simulink model "HW_1_v2_2019a_signal_builder"  (R2019a)
settings: Solver=VariableStepAuto  StartTime=0.0  StopTime=70  RelTol=1e-12
model workspace (MAT data in the model file):
  d_tar = 20
values from neighbouring files (symbols this model uses):
  d_0 = 8    [acc1.m]
  t_H_tar = 1    [acc1.m]
  v_H0 = 28    [acc1.m]
  v_L0 = 36    [acc1.m]
  v_tar = 36    [acc1.m]
  x_H0 = 0    [acc1.m]
  x_L0 = 50    [acc1.m]
undefined symbols (not defined in the file or in its folder): sigbuilder_block
libraries: cstblocks x3, fl_lib x1
settings Model: Creator=jake  LastModifiedBy=jake
settings DebuggingCC: SFMachineParentedDataDiag=error

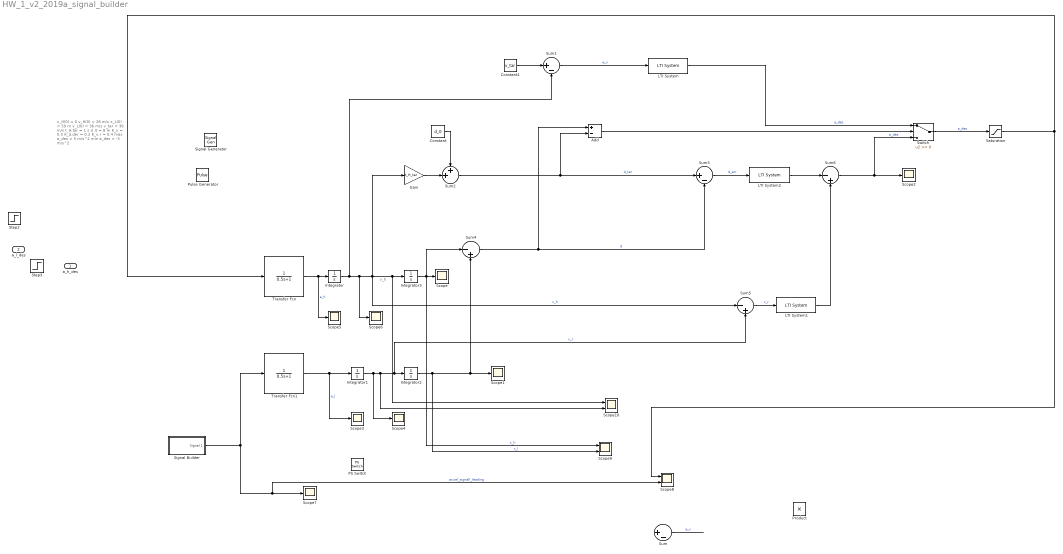
== system HW_1_v2_2019a_signal_builder ==
  note: x_H(0) = 0
      | v_H(0) = 28 m/s
      |
      | x_L(0) = 50 m
      | v_L(0) = 36 m/s
      |
      | v_tar = 36 m/s
      | t_H,tar = 1 s
      | d_0 = 8 m
      |
      | K_v = 0.5
      | K_d,der = 0.2
      | K_v,r = 0.4
      |
      | max a_des = 5 m/s^2
      | min a_des = -3 m/s^2
  note: v_h
  a_h_des : Inport
  a_l_des : Inport  Port=2
  Add : Sum  Inputs=+-
  Constant : Constant  Value=d_0
  Constant1 : Constant  Value=v_tar
  Gain : Gain  Gain=t_H_tar
  Integrator : Integrator  InitialCondition=v_H0
  Integrator1 : Integrator  InitialCondition=v_L0
  Integrator2 : Integrator  InitialCondition=x_L0
  Integrator3 : Integrator  InitialCondition=x_H0
  LTI System : cstblocks/LTI System  sys=K_v  IC=[]
  LTI System1 : cstblocks/LTI System  sys=K_v_r  IC=[]
  LTI System2 : cstblocks/LTI System  sys=K_d_err  IC=[]
  PS Switch : fl_lib/Physical Signals/Nonlinear Operators/PS Switch  Threshold=0.5
      settings: SourceProductBaseCode=SS  InternalSimscapePortConfiguration="{\"Bottom\":[],\"Left\":[{\"id\":\"I1\",\"label\":\"\",\"type\":\"input\"},{\"id\":\"I2\",\"label\":\"\",\"type\":\"input\"},{\"id\":\"I3\",\"label\":\"\",\"type\":\"input\"}],\"Right\":[{\"id\":\"O\",\"label\":\"\",\"type\":\"output\"}],\"Top\":[]}"
  Product : Product
  Pulse Generator : DiscretePulseGenerator  PulseType=Time based  Period=10  PulseWidth=5
  Saturation : Saturate  UpperLimit=5  LowerLimit=-3
  Scope{,1..7} (8 alike) : Scope
  Scope10 : Scope  NumInputPorts=2
  Scope8 : Scope  NumInputPorts=2
  Scope9 : Scope  NumInputPorts=2
  Signal Generator : SignalGenerator  Units=rad/sec
  Signal Builder : Subsystem  Tag=STV Subsys  LoadFcn=sigbuilder_block('load');  StartFcn=sigbuilder_block('start');  StopFcn=sigbuilder_block('stop');  ClipboardFcn=sigbuilder_block('clipboard');  mask(Sigbuilder block){tuvar=[0:10]}
      mask help: Simulink:masks:SigbuilderBlock_MD
      mask init:
      | if ~strcmp(get_param(bdroot(gcbh),'SimulationStatus'),'stopped') tuvar = sigbuilder_block('maskInit'); end
      settings: CopyFcn=sigbuilder_block('copy');  DeleteFcn=sigbuilder_block('delete');  ModelCloseFcn=sigbuilder_block('modelClose');  PreSaveFcn=sigbuilder_block('preSave');  PauseFcn=sigbuilder_block('pause');  ContinueFcn=sigbuilder_block('continue');  NameChangeFcn=sigbuilder_block('namechange');  OpenFcn=sigbuilder_block('open',[553.5 167.25 843.75 498.75 ]);  CloseFcn=sigbuilder_block('close');
      mask Display: plot(0, 0, 100, 100,[2, 2, 32, 32, 2], [68, 8, 8, 68, 68],[32, 2], [38, 38], [32, 19, 2],[53, 60, 44], [32, 17, 17, 2],[16, 16, 31, 31]);txt = getActiveGroup(gcbh);text(2, 100, txt,'verticalAlignment', 'top');
  Step2 : Step  Time=40  After=2  SampleTime=0
  Step3 : Step  Time=43.5  After=-2  SampleTime=0
  Sum : Sum  Inputs=|+-
  Sum1 : Sum  Inputs=|+-
  Sum2 : Sum  Inputs=++|
  Sum3 : Sum  Inputs=|+-
  Sum4 : Sum  Inputs=|-+
  Sum5 : Sum  Inputs=|-+
  Sum6 : Sum  Inputs=|-+
  Switch : Switch
  Transfer Fcn : TransferFcn  Denominator=[0.5 1]
  Transfer Fcn1 : TransferFcn  Denominator=[0.5 1]
  wires:
  Transfer Fcn/1 -> Scope5/1, Integrator/1  "a_h"
  Transfer Fcn1/1 -> Scope3/1, Integrator1/1  "a_l"
  Integrator1/1 -> Scope4/1, Scope10/2, Sum5/2, Integrator2/1  "v_l"
  Integrator/1 -> Sum1/2, Scope6/1, Sum5/1, Scope10/1, Integrator3/1, Gain/1  "v_h"
  Integrator2/1 -> Scope9/2, Scope1/1, Sum4/2  "x_l"
  Integrator3/1 -> Scope9/1, Sum4/1, Scope/1  "x_h"
  ? -> Sum/1  "v_tar"
  ? -> Sum/2  "v_h"
  Sum/1 -> ?  "e_v"
  Sum1/1 -> LTI System/1  "e_v"
  Gain/1 -> Sum2/2
  Constant/1 -> Sum2/1
  Sum2/1 -> Add/2, Sum3/1  "d_tar"
  Sum4/1 -> Add/1, Sum3/2  "d"
  Sum5/1 -> LTI System1/1  "v_r"
  Sum3/1 -> LTI System2/1  "d_err"
  LTI System1/1 -> Sum6/2
  LTI System2/1 -> Sum6/1
  Sum6/1 -> Switch/3, Scope2/1  "a_des"
  LTI System/1 -> Switch/1  "a_des"
  Constant1/1 -> Sum1/1
  Switch/1 -> Saturation/1  "a_des"
  Signal Builder/1(Signal 1) -> Scope8/2, Scope7/1, Transfer Fcn1/1  "accel_signall_leading"
  Saturation/1 -> Scope8/1, Transfer Fcn/1
  Add/1 -> Switch/2

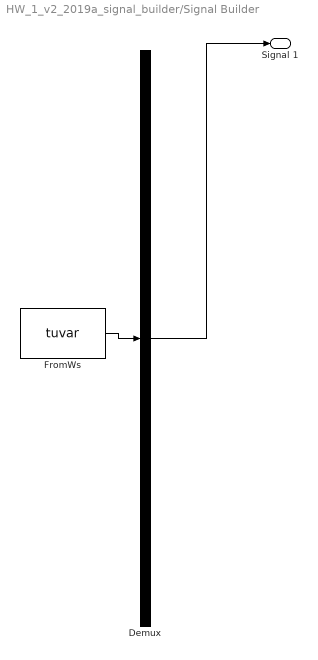
== system HW_1_v2_2019a_signal_builder/Signal Builder ==
  Demux : Demux  Tag=STV Demux  Outputs=1
      settings: DisplayOption=none
  FromWs : FromWorkspace  Tag=STV FromWs  VariableName=tuvar
      SigBuilderData=|
      | common.afterFinalStr = 'Extrapolate'
      | common.sampleTime = 0
      | dataSet.timeRange = [0 46]
      | dataSet.name = 'Group 1'
      | sbobj.Groups.Name = 'Group 1'
      | sbobj.Groups.Signals.Name = 'Signal 1'
      | sbobj.Groups.Signals.XData = [0 10 10.5 13.5 14 40 40.5 43.5 44 46]
      | sbobj.Groups.Signals.YData = [0 0 -2 -2 0 0 2 2 0 0.02]
      | sbobj.Groups.TimeRange = [0 46]
  Signal 1 : Outport  Tag=STV Outport
  wires:
  Demux/1 -> Signal 1/1
  FromWs/1 -> Demux/1
